simulink model "chap8_2sim"  (Simulink 7.7)
settings: Solver=ode45  StartTime=0.0  StopTime=10  RelTol=1e-3
settings Model: Creator=ljk  LastModifiedBy=ljk  ExtModeTrigMode=oneshot  ExtModeArmWhenConnect=off
settings DataIOCC: LimitDataPoints=off  SignalLoggingName=sigsOut
settings OptimizationCC: BooleanDataType=off
settings DebuggingCC: SaveWithParameterizedLinksMsg=none  SignalResolutionControl=TryResolveAllWithWarning  SolverPrmCheckMsg=none  MultiTaskDSMMsg=warning  MultiTaskCondExecSysMsg=none  StrictBusMsg=None
settings HardwareCC: TargetUnknown=on
settings RTWCC: IncludeERTFirstTime=on

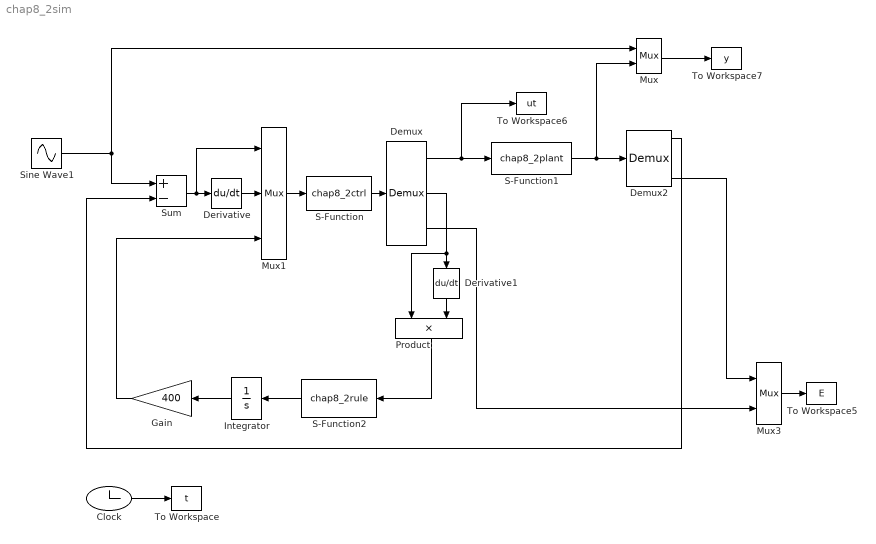
== system chap8_2sim ==
  Clock : Clock
  Demux : Demux  Outputs=3
  Demux2 : Demux  Outputs=3
  Derivative : Derivative
  Derivative1 : Derivative
  Gain : Gain  Gain=400  SaturateOnIntegerOverflow=on  OutDataTypeStr=Inherit: Same as input  ParamDataTypeStr=Inherit: Same as input
  Integrator : Integrator
  Mux : Mux  Inputs=2
  Mux1 : Mux  Inputs=3
  Mux3 : Mux  Inputs=2
  Product : Product  SaturateOnIntegerOverflow=on  InputSameDT=on  OutDataTypeStr=Inherit: Same as first input
  S-Function : S-Function  FunctionName=chap8_2ctrl  EnableBusSupport=off
  S-Function1 : S-Function  FunctionName=chap8_2plant  EnableBusSupport=off
  S-Function2 : S-Function  FunctionName=chap8_2rule  EnableBusSupport=off
  Sine Wave1 : Sin  Frequency=2*pi  SampleTime=0
  Sum : Sum  Inputs=+-  SaturateOnIntegerOverflow=on  InputSameDT=on  OutDataTypeStr=Inherit: Same as first input
  To Workspace : ToWorkspace  VariableName=t  SampleTime=-1  SaveFormat=Array
  To Workspace5 : ToWorkspace  VariableName=E  SampleTime=-1  SaveFormat=Array
  To Workspace6 : ToWorkspace  VariableName=ut  SampleTime=-1  SaveFormat=Array
  To Workspace7 : ToWorkspace  VariableName=y  SampleTime=-1  SaveFormat=Array
  wires:
  Mux1/1 -> S-Function/1
  S-Function/1 -> Demux/1
  Demux/2 -> Derivative1/1, Product/1
  Demux/1 -> S-Function1/1, To Workspace6/1
  S-Function1/1 -> Demux2/1, Mux/2
  Derivative/1 -> Mux1/2
  Sum/1 -> Mux1/1, Derivative/1
  Demux2/1 -> Sum/2
  Demux/3 -> Mux3/2
  S-Function2/1 -> Integrator/1
  Gain/1 -> Mux1/3
  Integrator/1 -> Gain/1
  Mux3/1 -> To Workspace5/1
  Mux/1 -> To Workspace7/1
  Product/1 -> S-Function2/1
  Clock/1 -> To Workspace/1
  Derivative1/1 -> Product/2
  Sine Wave1/1 -> Sum/1, Mux/1
  Demux2/3 -> Mux3/1
